simulink model "uloha7"  (Simulink 7.5)
settings: Solver=ode45  StartTime=0.0  StopTime=50.0  RelTol=1e-3
settings Model: Creator=michal  LastModifiedBy=michal

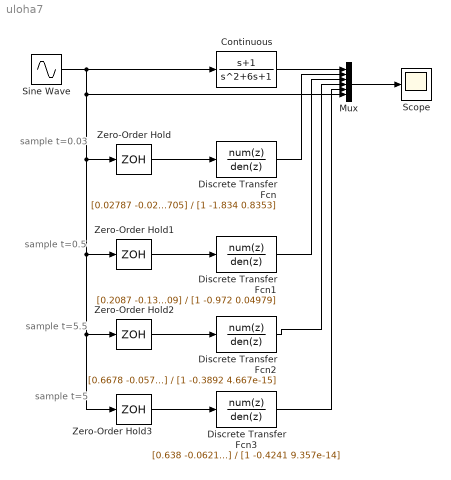
== system uloha7 ==
  note: sample t=0.03
  note: sample t=0.5
  note: sample t=5.5
  note: sample t=5
  Continuous : TransferFcn  Numerator=[1 1]  Denominator=[1 6 1]
  Discrete Transfer Fcn : DiscreteTransferFcn  Numerator=[0.02787 -0.02705]  Denominator=[1 -1.834 0.8353]  SampleTime=0.03
  Discrete Transfer Fcn1 : DiscreteTransferFcn  Numerator=[0.2087 -0.1309]  Denominator=[1 -0.972 0.04979]  SampleTime=0.5
  Discrete Transfer Fcn2 : DiscreteTransferFcn  Numerator=[0.6678 -0.057]  Denominator=[1 -0.3892 4.667e-15]  SampleTime=5.5
  Discrete Transfer Fcn3 : DiscreteTransferFcn  Numerator=[0.638 -0.0621]  Denominator=[1 -0.4241 9.357e-14]  SampleTime=5
  Mux : Mux  Inputs=6
  Scope : Scope
      settings: SaveName=data  DataFormat=Array
  Sine Wave : Sin  Amplitude=1  Bias=0  Frequency=3.141  Phase=0  Samples=1  SampleTime=0  Offset=0
  Zero-Order Hold : ZeroOrderHold  SampleTime=0.03
  Zero-Order Hold1 : ZeroOrderHold  SampleTime=0.5
  Zero-Order Hold2 : ZeroOrderHold  SampleTime=5.5
  Zero-Order Hold3 : ZeroOrderHold  SampleTime=5
  wires:
  Mux/1 -> Scope/1
  Continuous/1 -> Mux/1
  Sine Wave/1 -> Continuous/1, Zero-Order Hold1/1, Zero-Order Hold3/1, Zero-Order Hold2/1, Zero-Order Hold/1, Mux/6
  Zero-Order Hold/1 -> Discrete Transfer Fcn/1
  Zero-Order Hold1/1 -> Discrete Transfer Fcn1/1
  Zero-Order Hold2/1 -> Discrete Transfer Fcn2/1
  Zero-Order Hold3/1 -> Discrete Transfer Fcn3/1
  Discrete Transfer Fcn/1 -> Mux/2
  Discrete Transfer Fcn1/1 -> Mux/3
  Discrete Transfer Fcn2/1 -> Mux/4
  Discrete Transfer Fcn3/1 -> Mux/5
